simulink model "sl_groundvehicleDynamics-Kagrenac"  (R2025a)
settings: Solver=ode45  StartTime=0.0  StopTime=2000  RelTol=1e-5  EnableMultiTasking=on
InitFcn:
  | mdl_robot;
undefined symbols (not defined in the file): Ordered_Waypoints, robot
libraries: simulink x4, mobileRoboticsLib x3, simulink_extras x2
settings Model: Creator=sriramn  LastModifiedBy=hunte
settings SolverCC: ZeroCrossAlgorithm=Adaptive  AlgebraicLoopSolver=TrustRegion
settings DataIOCC: LimitDataPoints=on  SaveFormat=Array  ReturnWorkspaceOutputs=off
settings OptimizationCC: ReuseModelBlockBuffer=off  LifeSpan=inf
settings DebuggingCC: SolverPrmCheckMsg=warning  UnconnectedInputMsg=warning  UnconnectedOutputMsg=warning  UnconnectedLineMsg=warning  AllowSymbolicDim=off  SFUnexpectedBacktrackingDiag=warning  SFNoUnconditionalDefaultTransitionDiag=warning  SFExecutionAtInitializationDiag=none  ArithmeticOperatorsInVariantConditions=warning
settings HardwareCC: ProdBitPerPointer=32.0  ProdBitPerSizeT=32.0  ProdBitPerPtrDiffT=32.0  ProdLargestAtomicFloat=None  ProdIntDivRoundTo=Undefined  ProdEndianess=Unspecified  ProdWordSize=32.0  ProdHWDeviceType=32-bit Generic
settings ModelReferenceCC: EnableRefExpFcnMdlSchedulingChecks=on  ModelReferenceMinAlgLoopOccurrences=on  PropagateSignalLabelsOutOfModel=off
settings SFSimCC: SimUseLocalCustomCode=off  CustomCodeUndefinedFunction=UseInterfaceOnly
settings RTWCC: RTWUseLocalCustomCode=off  GPUComputeCapability=3.5
settings CodeAppCC: StateflowObjectComments=on
settings GRTTargetCC: TargetLangStandard=C89/C90 (ANSI)
settings ConfigComp: CovMetricSettings=dw  CovSaveCumulativeToWorkspaceVar=on  CovSaveSingleToWorkspaceVar=on  CovExternalEMLEnable=off  CovSFcnEnable=off
settings SimscapeCC: SimscapeNormalizeSystem=off
settings ConfigurationSet: Description=SimMechanics 2G
settings ExplorerConfigSet: InternalSimMechanicsExplorerSettings="<ExplorerConfiguration><canonicalview>planar_xy</canonicalview><AnimationSetting><BasePlaybackSpeed>1.0</BasePlaybackSpeed><PlaybackSpeedFactor>1.0</PlaybackSpeedFactor></AnimationSetting><TilePanel><TileInfo><Tiles Columns=\"1\" Count=\"1\" Rows=\"1\"><Column Left=\"2\" Weight=\"1\"/><Column Left=\"1628\"/><Row Top=\"2\" Weight=\"1\"/><Row Top=\"1072\"/><Tile Height=\"1\" Width=\"1\" X=\"0\" Y=\"0\"/></Tiles></TileInfo><SceneInfo><SceneViewer><BGColor><R>0.60000002384185791</R><G>0.60000002384185791</G><B>0.60000002384185791</B></BGColor><Camera><Position><X>0.22951840878551699</X><Y>0.32651610611526627</Y><Z>-0.27215421354393321</Z></Position><Center><X>-0.15775714411666431</X><Y>-0.15462825985839526</Y><Z>0.065702552916005602</Z></Center><Up><X>-0.56030137557930915</X><Y>0.72817587161684794</Y><Z>0.39474329445726858</Z></Up><Left>-0.21481383955700509</Left><Right>0.21481383955700509</Right><Bottom>-0.27569784609469139</Bottom><Top>0.27569784609469139</Top></Camera></SceneViewer></SceneInfo></TilePanel></ExplorerConfiguration>"

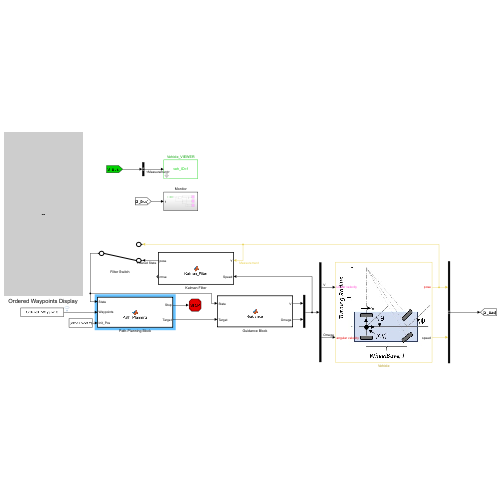
[thumbnail: Simulink's stored preview of the top-level diagram]
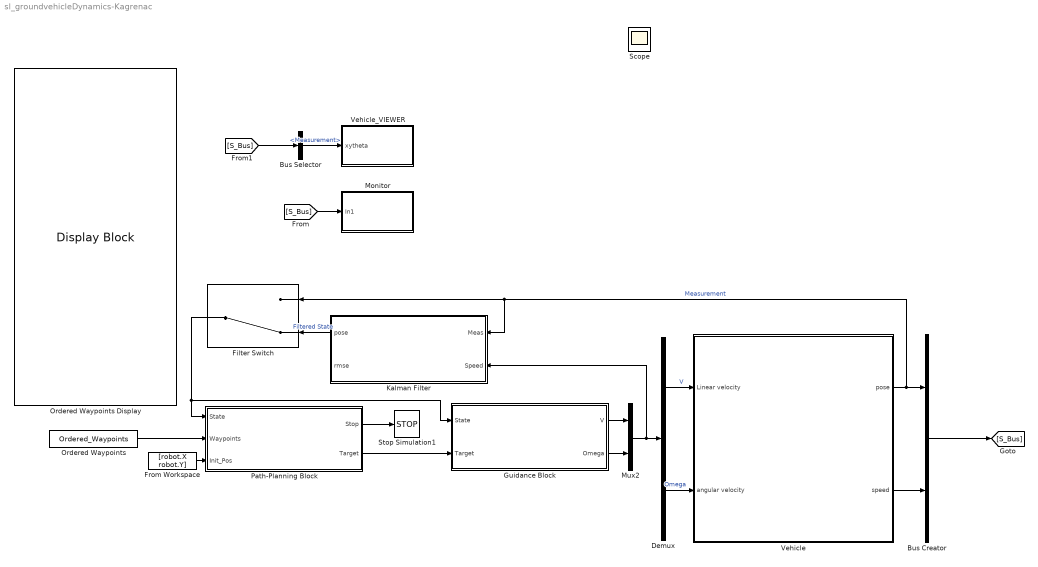
== system sl_groundvehicleDynamics-Kagrenac ==
  Bus Creator : BusCreator  Inputs=2
  Bus Selector : BusSelector  OutputSignals=Measurement
  Demux : Demux  Outputs=2
  Filter Switch : ManualSwitch  CurrentSetting=0
  From Workspace : FromWorkspace  VariableName=[robot.X robot.Y]  Interpolate=off  ZeroCross=off
  Guidance Block : MATLAB Function  TreatAsAtomicUnit=on
  Kalman Filter : MATLAB Function  TreatAsAtomicUnit=on
  Monitor : Subsystem
  Mux2 : Mux  Inputs=2
  Ordered Waypoints : Constant  Value=Ordered_Waypoints  VectorParams1D=off
  Ordered Waypoints Display : DisplayBlock  LabelPosition=Hide  Transparency=1  GridColor=[0.502, 0.502, 0.502]
  Path-Planning Block : MATLAB Function  TreatAsAtomicUnit=on
  Stop Simulation1 : Stop
  Vehicle : Subsystem
      mask Display: image('vehicle.jpg');
  Vehicle_VIEWER : Subsystem  mask{wp_mat=[-500, 500; -500, 500]', veh_ID_num=1, veh_init_xytheta=[robot.X robot.Y robot.Theta], Ts=0.5}
      mask prompts: wp_mat "Waypoint matrix for arena [x_col, y_col] (m)"; veh_ID_num "Vehicle ID number"; veh_init_xytheta "Initial pose [x,y,theta]"; Ts "Sample time for updating animation (secs)"
      mask TypeOptions veh_ID_num: 1 | 2 | 3 | 4
      mask DialogControl Control2 Prompt: Animate simulation of Differential Drive Robot (DDR)
      mask Display: fprintf('veh_ID=%d',veh_ID_num);
  Scope : Scope
      settings: ActiveDisplayYMinimum=0.07  ActiveDisplayYMaximum=0.09
  wires:
  [S_Bus] -> Monitor/1(In1)
  [S_Bus] -> Bus Selector/1
  Vehicle/2(speed) -> Bus Creator/2
  Bus Creator/1 -> [S_Bus]
  Bus Selector/1 -> Vehicle_VIEWER/1(xytheta)  "<Measurement>"
  Filter Switch/1 -> Path-Planning Block/1(State), Guidance Block/1(State)
  Demux/1 -> Vehicle/1(Linear velocity)  "V"
  Guidance Block/1(V) -> Mux2/1
  Guidance Block/2(Omega) -> Mux2/2
  Demux/2 -> Vehicle/2(angular velocity)  "Omega"
  Mux2/1 -> Kalman Filter/2(Speed), Demux/1
  Path-Planning Block/2(Target) -> Guidance Block/2(Target)
  Ordered Waypoints/1 -> Path-Planning Block/2(Waypoints)
  Vehicle/1(pose) -> Bus Creator/1, Kalman Filter/1(Meas), Filter Switch/1  "Measurement"
  Kalman Filter/1(pose) -> Filter Switch/2  "Filtered State"
  Path-Planning Block/1(Stop) -> Stop Simulation1/1
  From Workspace/1 -> Path-Planning Block/3(Init_Pos)

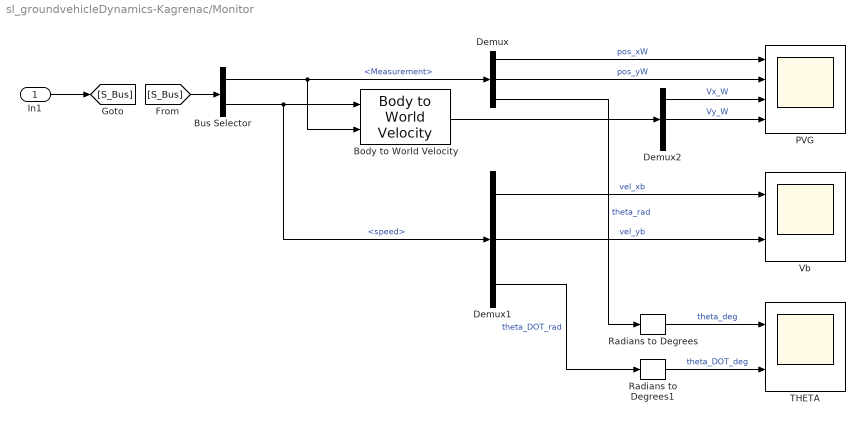
== system sl_groundvehicleDynamics-Kagrenac/Monitor ==
  In1 : Inport
  Body to World Velocity : mobileRoboticsLib/Utilities/Body to World Velocity
      settings: SourceProductName=Mobile Robotics Simulation Toolbox
  Bus Selector : BusSelector  OutputSignals=Measurement,speed
  Demux : Demux  Outputs=3
  Demux1 : Demux  Outputs=3
  Demux2 : Demux  Outputs=3
  PVG : Scope  NumInputPorts=4
      settings: ActiveDisplayYMinimum=-3.02358  ActiveDisplayYMaximum=27.35477
  Radians to Degrees : simulink_extras/Transformations/Radians to Degrees
  Radians to Degrees1 : simulink_extras/Transformations/Radians to Degrees
  THETA : Scope  NumInputPorts=2
      settings: ActiveDisplayYMinimum=-8.72937  ActiveDisplayYMaximum=60.06611  DataLoggingVariableName=ScopeData2
  Vb : Scope  NumInputPorts=2
      settings: ActiveDisplayYMinimum=0.05577  ActiveDisplayYMaximum=0.8929
  wires:
  In1/1 -> [S_Bus]
  [S_Bus] -> Bus Selector/1
  Demux/1 -> PVG/1  "pos_xW"
  Demux/2 -> PVG/2  "pos_yW"
  Radians to Degrees1/1 -> THETA/2  "theta_DOT_deg"
  Radians to Degrees/1 -> THETA/1  "theta_deg"
  Demux1/3 -> Radians to Degrees1/1  "theta_DOT_rad"
  Demux/3 -> Radians to Degrees/1  "theta_rad"
  Bus Selector/1 -> Body to World Velocity/2, Demux/1  "<Measurement>"
  Bus Selector/2 -> Demux1/1, Body to World Velocity/1  "<speed>"
  Body to World Velocity/1 -> Demux2/1
  Demux2/1 -> PVG/3  "Vx_W"
  Demux2/2 -> PVG/4  "Vy_W"
  Demux1/1 -> Vb/1  "vel_xb"
  Demux1/2 -> Vb/2  "vel_yb"

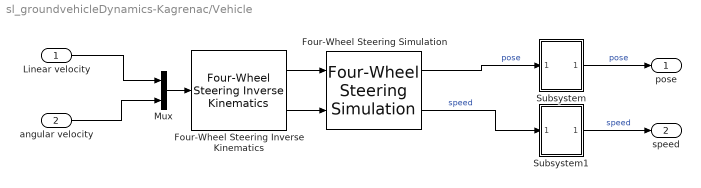
== system sl_groundvehicleDynamics-Kagrenac/Vehicle ==
  Linear velocity : Inport
  angular velocity : Inport  Port=2
  Four-Wheel Steering Inverse Kinematics : mobileRoboticsLib/Kinematic Models/Four-Wheel Steering/Four-Wheel Steering Inverse Kinematics  wheelRadius=0.1  frontWheelDist=0.25  rearWheelDist=0.25  ikMode=Front Steering
      settings: SourceProductName=Mobile Robotics Simulation Toolbox
  Four-Wheel Steering Simulation : mobileRoboticsLib/Kinematic Models/Four-Wheel Steering/Four-Wheel Steering Simulation  wheelRadius=0.1  frontWheelDist=0.25  rearWheelDist=0.25  initX=robot.X  initY=robot.Y  initAngle=robot.Theta  Ts=0.05
      settings: SourceProductName=Mobile Robotics Simulation Toolbox
  Mux : Mux  Inputs=2
  Subsystem : Subsystem
  Subsystem1 : Subsystem
  pose : Outport  VectorParamsAs1DForOutWhenUnconnected=off
  speed : Outport  Port=2
  wires:
  angular velocity/1 -> Mux/2
  Linear velocity/1 -> Mux/1
  Mux/1 -> Four-Wheel Steering Inverse Kinematics/1
  Four-Wheel Steering Simulation/1 -> Subsystem/1(In1)  "pose"
  Four-Wheel Steering Simulation/2 -> Subsystem1/1(In1)  "speed"
  Four-Wheel Steering Inverse Kinematics/1 -> Four-Wheel Steering Simulation/1
  Four-Wheel Steering Inverse Kinematics/2 -> Four-Wheel Steering Simulation/2
  Subsystem/1(pose) -> pose/1  "pose"
  Subsystem1/1(speed) -> speed/1  "speed"

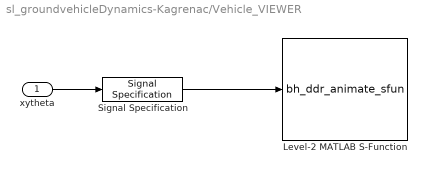
== system sl_groundvehicleDynamics-Kagrenac/Vehicle_VIEWER ==
  xytheta : Inport
  Level-2 MATLAB S-Function : M-S-Function  FunctionName=bh_ddr_animate_sfun  Parameters=Ts, Ordered_Waypoints, veh_ID_num, veh_init_xytheta
  Signal Specification : SignalSpecification  Dimensions=3
  wires:
  xytheta/1 -> Signal Specification/1
  Signal Specification/1 -> Level-2 MATLAB S-Function/1

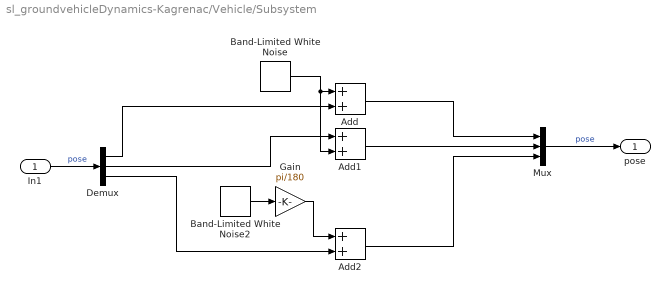
== system sl_groundvehicleDynamics-Kagrenac/Vehicle/Subsystem ==
  In1 : Inport
  Add : Sum
  Add1 : Sum
  Add2 : Sum
  Band-Limited White Noise : simulink/Sources/Band-Limited White Noise  Cov=[0.001]  Ts=0.1  seed=[23341]
  Band-Limited White Noise2 : simulink/Sources/Band-Limited White Noise  Cov=[0.41]  Ts=0.1  seed=[23341]
  Demux : Demux  Outputs=3
  Gain : Gain  Gain=pi/180
  Mux : Mux  Inputs=3
  pose : Outport
  wires:
  Add1/1 -> Mux/2
  Add2/1 -> Mux/3
  Demux/2 -> Add1/1
  Band-Limited White Noise2/1 -> Gain/1
  Demux/3 -> Add2/2
  Band-Limited White Noise/1 -> Add1/2, Add/1
  In1/1 -> Demux/1  "pose"
  Demux/1 -> Add/2
  Gain/1 -> Add2/1
  Mux/1 -> pose/1  "pose"
  Add/1 -> Mux/1

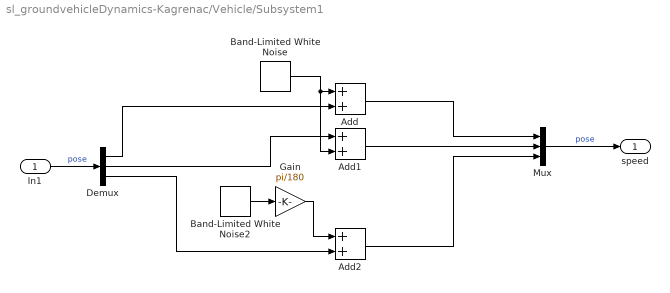
== system sl_groundvehicleDynamics-Kagrenac/Vehicle/Subsystem1 ==
  In1 : Inport
  Add : Sum
  Add1 : Sum
  Add2 : Sum
  Band-Limited White Noise : simulink/Sources/Band-Limited White Noise  Cov=[0.001]  Ts=0.1  seed=[23341]
  Band-Limited White Noise2 : simulink/Sources/Band-Limited White Noise  Cov=[0.41]  Ts=0.1  seed=[23341]
  Demux : Demux  Outputs=3
  Gain : Gain  Gain=pi/180
  Mux : Mux  Inputs=3
  speed : Outport
  wires:
  Add1/1 -> Mux/2
  Add2/1 -> Mux/3
  Demux/2 -> Add1/1
  Band-Limited White Noise2/1 -> Gain/1
  Demux/3 -> Add2/2
  Band-Limited White Noise/1 -> Add1/2, Add/1
  In1/1 -> Demux/1  "pose"
  Demux/1 -> Add/2
  Gain/1 -> Add2/1
  Mux/1 -> speed/1  "pose"
  Add/1 -> Mux/1

== matlab function sl_groundvehicleDynamics-Kagrenac/Path-Planning Block ==
  data: Stop output; Target output; State input; Waypoints input; Init_Pos input
function [Stop, Target] = Path_Planning(State, Waypoints, Init_Pos)


persistent WP_List;
persistent N_WPs;
persistent Target_WP_Idx;


Stop = 0;


%% Configs:

% Distance from WP that Counts as Visited:
WP_Thresh = 10;

% How Far Forward the RVWP should be from the Robot's Projected Position:
LookAhead = 20;


% X-Y Position of the Robot:
Pos = [State(1), State(2)];


%% Parsing and Initialisation of Waypoints:

if isempty(WP_List)

    N_WPs = size(Waypoints, 1);

    WP_List = repmat(struct("Pos", zeros(1, 2), "Visited", false, "Vect", zeros(1, 2), "Len", 0, "Dir", zeros(1, 2)), 1, N_WPs);

    % Turning the List of WPs into a Struct Array:
    for k = 1:N_WPs

        WP_List(k).Pos = Waypoints(k, :);

        if k ~= 1,  WP_List(k).Vect = Waypoints(k, :) - Waypoints(k-1, :);
        else,       WP_List(k).Vect = Waypoints(k, :) - Init_Pos;
        end

        WP_List(k).Len = norm(WP_List(k).Vect);
        WP_List(k).Dir = WP_List(k).Vect / WP_List(k).Len;
    
    end

    Target_WP_Idx = 1;
end


%% Indexing Target WP:

if sqrt( (WP_List(Target_WP_Idx).Pos(1)-State(1))^2 + (WP_List(Target_WP_Idx).Pos(2)-State(2))^2 ) < WP_Thresh

    WP_List(Target_WP_Idx).Visited = true;

    if (Target_WP_Idx == N_WPs), Stop = 1;
    else, Target_WP_Idx = Target_WP_Idx + 1;
    end

end


%% Calculating Vector Projection onto Segment + LookAhead:


Dot_Product_Proj =  dot(WP_List(Target_WP_Idx).Vect, (Pos - WP_List(Target_WP_Idx).Pos)) / WP_List(Target_WP_Idx).Len;

Target = WP_List(Target_WP_Idx).Pos + ((Dot_Product_Proj + LookAhead) * WP_List(Target_WP_Idx).Dir);

== matlab function sl_groundvehicleDynamics-Kagrenac/Kalman Filter ==
  data: Meas input; pose output; rmse output; Speed input
function [pose, rmse] = Kalman_Filter(Meas, Speed)
%{
Argument Shapes:
Constants =   [Q      R]
IN:
    Meas    = [Pos_x    Pos_y   Theta] % Unfiltered state measurement
    Speed   = [V        Omega]         % Control input
OUT:
    X       = [Pos_x    Pos_y   Theta   V_x V_y Omega] % Filtered/Estimated state
    pose    = [Pos_x    Pos_y   Theta] % Subset of X
%}

%% Model Declaration [X], [U], [Y], [P]
% Extract measurements
Pos_x = Meas(1); Pos_y = Meas(2); Theta = Meas(3);

% Control Input [U]
V_x = Speed(1) * cos(Theta); V_y = Speed(1) * sin(Theta); Omega = Speed(2);
U = [0 0 0 V_x V_y Omega]'; % Controlling velocity states, not positional states
%{
Transpose `U` to eliminate the need for `B`, such that ...
Pos:    x(k)    = x(k-1) + x_dot(k-1)*dt
Speed:  x_dot(k)= x_dot(k-1) + u(k-1)
%}

% Vehicle Output [Y]
Y = [Pos_x Pos_y Theta 0 0 0]'; % Measuring positional states, not velocity states

% Model State [X] & Variance [P]
persistent X P k
if isempty(X)
    X = [Pos_x Pos_y Theta V_x V_y Omega]'; % [X; X_dot]
    P = 10 * eye(6);
    k = 1; % first iteration
end

%% Initialise Filter Parameters
dt = 0.05;              % Time step
sim_len = 5000;         % Number of iterations
state_len = size(X, 1); % Number of states

% Variance from process noise
sigma_x = 0.1; sigma_y = 0.1; sigma_theta = deg2rad(2);

% Variance from measurement noise
sigma_q = 1e-2;

% Covariance matrices
Q = sigma_q * eye(state_len);                   % Process noise (X)
R = diag([sigma_x sigma_y sigma_theta 0 0 0]);  % Measurement noise (Y)

% State-space matrices
A = eye(state_len); % Initialise such that Pos_x(k) = Pos_x(k-1), etc.
A(1,4) = dt;        % Substitute such that Pos_x(k) = Pos_x(k-1) + V_x*dt ...
A(2,5) = dt;        % ... Pos_y(k) = Pos_y(k-1) + V_y*dt ...
A(3,6) = dt;        % ... Theta(k) = Theta(k-1) + Omega*dt

H = diag([1 1 1 0 0 0]); % Measure only positional states

% Store corrected values for each time step
X_arr = zeros(state_len, sim_len);  % States
% P_arr = zeros(state_len, sim_len);  % Error covariances
% K_arr = zeros(state_len, sim_len);  % Kalman gains

X_arr(:,1) = X; % P_arr(:,1) = P;     % Store initial values

%% Filtering
% Update predictions
X_predict = X + B * U;      % X(k) = X(k-1) + B * U(k)
P_predict = P + Q; % P(k) = P(k-1) + Q

% Correct predictions from measurement
K_k = P_predict * H' / (H * P_predict * H'+ R);
X = X_predict + K_k * (Y - H * X_predict);
P = (eye(stat_len) - K_k * H) * P_predict;

X_arr(:,k) = X; % Store states for RMSE calculation

% Currently not needed
%{
for i = 1:stat_len
    % Store kalman gains
    K_arr(i,k) = K_k(i,1);

    % Store error covariance values
    P_arr(i,k) = P(i,1);
end
%}

%% Outputs
% Filtered positional states
pose = X(1:3)';

% Root Mean Squared Error
if k == sim_len % only calculate on the last iteration
    e = Meas' - X_arr(1,:)';
    rmse = 1 / rms(e(:,1));
end

k = k + 1; % Count the number of iterations

end

== matlab function sl_groundvehicleDynamics-Kagrenac/Guidance Block ==
  data: State input; V output; Omega output; Target input
function [V, Omega] = Guidance(State, Target)

persistent Last_Delta;
persistent Last_RTP;


%% Configs:

    
V   = 1.5;      % Constant Velocity (V),    (Originally [v = 0.99])
Kp  = 0.1;      % Proportional Gain (Kp),   (Originally [0.8])
Kd  = 0.1;      % Derivative Gain   (Kd),   (Originally [0.8])
N   = 4.0;      % Navigation Gain   (N),    (Ideally [3<=N<=5])


%% Range and Heading:

% Flight Path Angle [Gamma], (rad):
Gamma = State(3);


% Relative Target Position [RTP] in the inertial frame, (m):
RTP = [(Target(1) - State(1));... % dx
    (Target(2) - State(2))];      % dy

% Range to Target [Range], (m):
Range = norm(RTP);

% Line-Of-Sight [Lambda] Angle, (rad):
Lambda = atan2(RTP(2),RTP(1));


%% Proportional [P] (Pure Pursuite):

% Heading Error [Delta], (rad):
Delta = Lambda - Gamma;
if      (Delta < -pi),  Delta = Delta + 2*pi;
elseif  (Delta > +pi),  Delta = Delta - 2*pi;
end


%% Derivitive [D] (Proportional Navigation):

t_step = 0.1;

if isempty(Last_Delta), Last_Delta  = Delta;   end
if isempty(Last_RTP),   Last_RTP    = RTP;     end

Delta_dot   = (Delta - Last_Delta) ./ t_step;                               % Delta_dot     - Heading Error Time Derivitive.
RTP_dot     = (RTP - Last_RTP) ./ t_step;                                   % RTP_dot       - Relative Target Position Time Derivitive.
Range_dot   = norm(RTP_dot);                                                % Range_dot     - Distance to Target Time Derivitive
Lambda_dot  = ( (RTP(1)*RTP_dot(2)) - (RTP(2)*RTP_dot(1)) ) / ( Range^2 );  % Lambda_dot    - LOS Angle Time Derivitive.

Last_Delta = Delta;
Last_RTP = RTP;



%% Controller Types:

% if (abs(Delta) > pi/3)
%     if (0)
%     Omega = (Kp * Delta);                                                   % [P] Controller (Pure Pursuit).
%     else
%     Omega = (Kp * Delta) + (Kd * Delta_dot);                                % [PD] Controller (Pure Pursuit).
%     end
% else
%     Omega = (N * Lambda_dot);                                               % [D] Controller (Proportional Navigation).
% end



%% Pure Pursuit:

Omega = (Kp * Delta) + (Kd * Delta_dot);                                    % [PD] Controller (Pure Pursuit).



%% Output Logging:

% LOS         = Lambda    * (180/pi);
% Heading     = Gamma     * (180/pi);
% Lead_Angle  = Delta     * (180/pi);
% 
% LoggingOutput = [LOS Heading Lead_Angle];
